simulink model "model"  (R2021a)
settings: Solver=VariableStepAuto  StartTime=0.0  StopTime=11  RelTol=1e-3
values from neighbouring files (symbols this model uses):
  b = .071    (= 0.071)    [main.m]
  Ipn = 2    [main.m]
  J = 21890.7e-6    (= 0.0218907)    [main.m]
  K = .573    (= 0.573)    [main.m]
  L = 5.4e-3    (= 0.0054)    [main.m]
  M = 171    [main.m]
  phi_max = 10    [main.m]
  R = 1.45    [main.m]
  Ts = 0.001    [main.m]
  U = 48    [main.m]
  U_I_max = 4    [main.m]
libraries: simulink x5, pid_lib x2, spsPWMGeneratorDCDCLib x1, eeQuadratureDecoder x1
settings Model: Creator=artof  LastModifiedBy=artof
settings SolverCC: AlgebraicLoopSolver=TrustRegion
settings DebuggingCC: SFMachineParentedDataDiag=warning

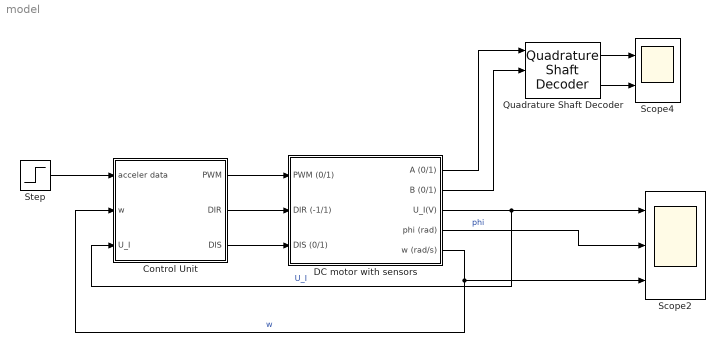
== system model ==
  Control Unit : Subsystem
  DC motor with sensors : Subsystem
  Quadrature Shaft Decoder : eeQuadratureDecoder/Quadrature Shaft Decoder  NPulse=4  Ts=Ts
      settings: SourceProductBaseCode=PS
  Scope2 : Scope  NumInputPorts=3
  Scope4 : Scope  NumInputPorts=2
  Step : Step  After=9.81  SampleTime=0
  wires:
  DC motor with sensors/1(A (0/1)) -> Quadrature Shaft Decoder/1
  DC motor with sensors/2(B (0/1)) -> Quadrature Shaft Decoder/2
  DC motor with sensors/5(w (rad/s)) -> Control Unit/2(w), Scope2/3  "w"
  DC motor with sensors/4(phi (rad)) -> Scope2/2  "phi"
  DC motor with sensors/3(U_I(V)) -> Scope2/1, Control Unit/3(U_I)  "U_I"
  Control Unit/1(PWM) -> DC motor with sensors/1(PWM (0/1))
  Control Unit/2(DIR) -> DC motor with sensors/2(DIR (-1/1))
  Control Unit/3(DIS) -> DC motor with sensors/3(DIS (0/1))
  Quadrature Shaft Decoder/1 -> Scope4/1
  Quadrature Shaft Decoder/2 -> Scope4/2
  Step/1 -> Control Unit/1(acceler data)

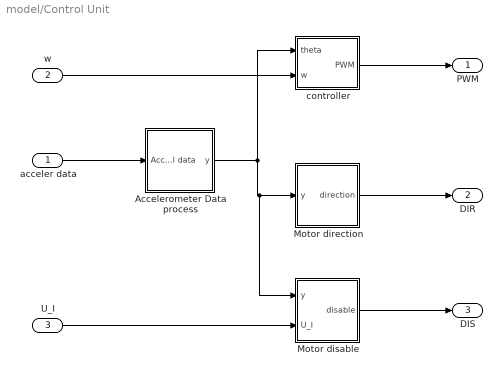
== system model/Control Unit ==
  acceler data : Inport
  w : Inport  Port=2
  U_I : Inport  Port=3
  Accelerometer Data process : Subsystem
  Motor direction : Subsystem
  Motor disable : Subsystem
  controller : Subsystem
  PWM : Outport
  DIR : Outport  Port=2
  DIS : Outport  Port=3
  wires:
  Accelerometer Data process/1(y) -> controller/1(theta), Motor disable/1(y), Motor direction/1(y)
  acceler data/1 -> Accelerometer Data process/1(Accel data)
  Motor direction/1(direction) -> DIR/1
  w/1 -> controller/2(w)
  controller/1(PWM) -> PWM/1
  U_I/1 -> Motor disable/2(U_I)
  Motor disable/1(disable) -> DIS/1

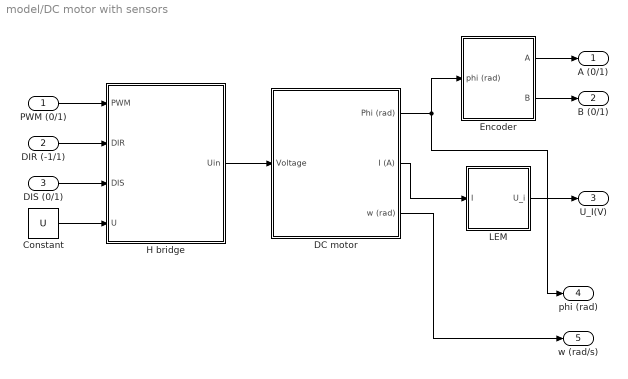
== system model/DC motor with sensors ==
  PWM (0/1) : Inport
  DIR (-1/1) : Inport  Port=2
  DIS (0/1) : Inport  Port=3
  Constant : Constant  Value=U
  DC motor : Subsystem
  Encoder : Subsystem
  H bridge : Subsystem
  LEM : Subsystem
  A (0/1) : Outport
  B (0/1) : Outport  Port=2
  U_I(V) : Outport  Port=3
  phi (rad) : Outport  Port=4
  w (rad/s) : Outport  Port=5
  wires:
  PWM (0/1)/1 -> H bridge/1(PWM)
  DIR (-1/1)/1 -> H bridge/2(DIR)
  H bridge/1(Uin) -> DC motor/1("Voltage ")
  DC motor/1(Phi (rad)) -> Encoder/1(phi (rad)), phi (rad)/1
  Encoder/2(B) -> B (0/1)/1
  Constant/1 -> H bridge/4(U)
  DC motor/2(I (A)) -> LEM/1(I)
  Encoder/1(A) -> A (0/1)/1
  LEM/1(U_i) -> U_I(V)/1
  DIS (0/1)/1 -> H bridge/3(DIS)
  DC motor/3(w (rad)) -> w (rad/s)/1

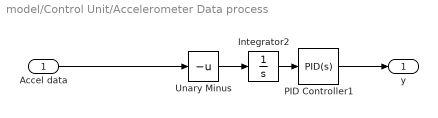
== system model/Control Unit/Accelerometer Data process ==
  Accel data : Inport
  Integrator2 : Integrator
  PID Controller1 : pid_lib/PID Controller  Controller=PID  Form=Parallel  TimeDomain=Continuous-time  UseExternalTs=off  SampleTime=-1  IntegratorMethod=Forward Euler  FilterMethod=Forward Euler  ControllerParametersSource=internal  P=1  I=0.1  D=0  UseFilter=on  N=100  TunerSelectOption=Transfer Function Based (PID Tuner App)  InitialConditionSource=internal  InitialConditionForIntegrator=0  InitialConditionForFilter=0  DifferentiatorICPrevScaledInput=0  ExternalReset=none  TrackingMode=off  Kt=1  LimitOutput=off  SatLimitsSource=internal  UpperSaturationLimit=inf  LowerSaturationLimit=-inf  LinearizeAsGain=on  AntiWindupMode=none  Kb=1  POutMin=[]  POutMax=[]  IOutMin=[]  IOutMax=[]  DOutMin=[]  DOutMax=[]  NOutMin=[]  NOutMax=[]  SumOutMin=[]  SumOutMax=[]  SaturationOutMin=[]  SaturationOutMax=[]  PParamMin=[]  PParamMax=[]  IParamMin=[]  IParamMax=[]  DParamMin=[]  DParamMax=[]  NParamMin=[]  NParamMax=[]  KbParamMin=[]  KbParamMax=[]  KtParamMin=[]  KtParamMax=[]  KbOutMin=[]  KbOutMax=[]  KtOutMin=[]  KtOutMax=[]  IntegratorOutMin=[]  IntegratorOutMax=[]  FilterOutMin=[]  FilterOutMax=[]  SumI1OutMin=[]  SumI1OutMax=[]  SumI2OutMin=[]  SumI2OutMax=[]  SumI3OutMin=[]  SumI3OutMax=[]  SumI4OutMin=[]  SumI4OutMax=[]  SumDOutMin=[]  SumDOutMax=[]  DifferentiatorOutMin=[]  DifferentiatorOutMax=[]  FilterDiffOutCoefMin=[]  FilterDiffOutCoefMax=[]  ReciprocalOutMin=[]  ReciprocalOutMax=[]  SumDenOutMin=[]  SumDenOutMax=[]  SumNumOutMin=[]  SumNumOutMax=[]  DivideOutMin=[]  DivideOutMax=[]  UdiffTsProdOutMin=[]  UdiffTsProdOutMax=[]  NTsProdOutMin=[]  NTsProdOutMax=[]  UintegralTsProdOutMin=[]  UintegralTsProdOutMax=[]  UngainTsProdOutMin=[]  UngainTsProdOutMax=[]  IntegratorContinuousStateAttributes=''  IntegratorStateMustResolveToSignalObject=off  IntegratorRTWStateStorageClass=Auto  FilterContinuousStateAttributes=''  FilterStateMustResolveToSignalObject=off  FilterRTWStateStorageClass=Auto  ParallelPVariant=InternalParameters  IdealPVariant=Disabled  IVariant=InternalParameters  DVariant=InternalParameters  IntegratorVariant=Continuous  SatVariant=Disabled  AWVariant=Passthrough  PCopyVariant=Disabled  TRVariant=Disabled  FdbkBlocksVariant=Forward  IdealPFdbkVariant=Disabled  SatFdbkVariant=Disabled  DerivativeFilterVariant=ContFilter  NVariant=InternalParameters  NCopyVariant=Disabled  FilterICVariant=InternalICsFilter  IntegratorICVariant=InternalICs  ExternalResetVariant=Disabled  TRSumVariant=Passthrough  SumFdbkVariant=Disabled  SumVariant=Sum_PID  TsampFilterVariant=InternalTs  TsampNgainVariant=Passthrough  TsampIntegralVariant=Passthrough  ExternalSaturationOutDataTypeStr=Inherit: Same as second input
  Unary Minus : UnaryMinus
  y : Outport
  wires:
  Integrator2/1 -> PID Controller1/1
  PID Controller1/1 -> y/1
  Unary Minus/1 -> Integrator2/1
  Accel data/1 -> Unary Minus/1

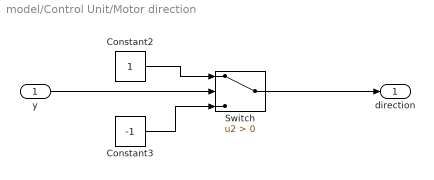
== system model/Control Unit/Motor direction ==
  y : Inport
  Constant2 : Constant
  Constant3 : Constant  Value=-1
  Switch : Switch  Criteria=u2 > Threshold
  direction : Outport
  wires:
  Constant3/1 -> Switch/3
  Switch/1 -> direction/1
  Constant2/1 -> Switch/1
  y/1 -> Switch/2

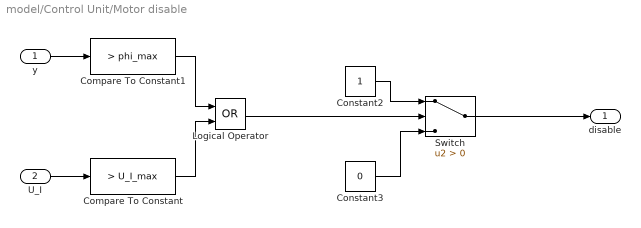
== system model/Control Unit/Motor disable ==
  y : Inport
  U_I : Inport  Port=2
  Compare To Constant : simulink/Logic and Bit Operations/Compare To Constant  relop=>  const=U_I_max  OutDataTypeStr=boolean
  Compare To Constant1 : simulink/Logic and Bit Operations/Compare To Constant  relop=>  const=phi_max  OutDataTypeStr=boolean
  Constant2 : Constant
  Constant3 : Constant  Value=0
  Logical Operator : Logic  Operator=OR  AllPortsSameDT=off  OutDataTypeStr=boolean
  Switch : Switch  Criteria=u2 > Threshold
  disable : Outport
  wires:
  Constant2/1 -> Switch/1
  Switch/1 -> disable/1
  Constant3/1 -> Switch/3
  U_I/1 -> Compare To Constant/1
  Compare To Constant/1 -> Logical Operator/2
  y/1 -> Compare To Constant1/1
  Compare To Constant1/1 -> Logical Operator/1
  Logical Operator/1 -> Switch/2

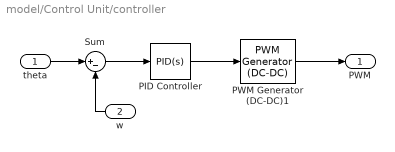
== system model/Control Unit/controller ==
  theta : Inport
  w : Inport  Port=2
  PID Controller : pid_lib/PID Controller  Controller=PID  Form=Parallel  TimeDomain=Continuous-time  UseExternalTs=off  SampleTime=-1  IntegratorMethod=Forward Euler  FilterMethod=Forward Euler  ControllerParametersSource=internal  P=100  I=0.1  D=0.001  UseFilter=on  N=100  TunerSelectOption=Transfer Function Based (PID Tuner App)  InitialConditionSource=internal  InitialConditionForIntegrator=0  InitialConditionForFilter=0  DifferentiatorICPrevScaledInput=0  ExternalReset=none  TrackingMode=off  Kt=1  LimitOutput=on  SatLimitsSource=internal  UpperSaturationLimit=1  LowerSaturationLimit=0  LinearizeAsGain=on  AntiWindupMode=none  Kb=1  POutMin=[]  POutMax=[]  IOutMin=[]  IOutMax=[]  DOutMin=[]  DOutMax=[]  NOutMin=[]  NOutMax=[]  SumOutMin=[]  SumOutMax=[]  SaturationOutMin=[]  SaturationOutMax=[]  PParamMin=[]  PParamMax=[]  IParamMin=[]  IParamMax=[]  DParamMin=[]  DParamMax=[]  NParamMin=[]  NParamMax=[]  KbParamMin=[]  KbParamMax=[]  KtParamMin=[]  KtParamMax=[]  KbOutMin=[]  KbOutMax=[]  KtOutMin=[]  KtOutMax=[]  IntegratorOutMin=[]  IntegratorOutMax=[]  FilterOutMin=[]  FilterOutMax=[]  SumI1OutMin=[]  SumI1OutMax=[]  SumI2OutMin=[]  SumI2OutMax=[]  SumI3OutMin=[]  SumI3OutMax=[]  SumI4OutMin=[]  SumI4OutMax=[]  SumDOutMin=[]  SumDOutMax=[]  DifferentiatorOutMin=[]  DifferentiatorOutMax=[]  FilterDiffOutCoefMin=[]  FilterDiffOutCoefMax=[]  ReciprocalOutMin=[]  ReciprocalOutMax=[]  SumDenOutMin=[]  SumDenOutMax=[]  SumNumOutMin=[]  SumNumOutMax=[]  DivideOutMin=[]  DivideOutMax=[]  UdiffTsProdOutMin=[]  UdiffTsProdOutMax=[]  NTsProdOutMin=[]  NTsProdOutMax=[]  UintegralTsProdOutMin=[]  UintegralTsProdOutMax=[]  UngainTsProdOutMin=[]  UngainTsProdOutMax=[]  IntegratorContinuousStateAttributes=''  IntegratorStateMustResolveToSignalObject=off  IntegratorRTWStateStorageClass=Auto  FilterContinuousStateAttributes=''  FilterStateMustResolveToSignalObject=off  FilterRTWStateStorageClass=Auto  ParallelPVariant=InternalParameters  IdealPVariant=Disabled  IVariant=InternalParameters  DVariant=InternalParameters  IntegratorVariant=Continuous  SatVariant=Enabled  AWVariant=Passthrough  PCopyVariant=Disabled  TRVariant=Disabled  FdbkBlocksVariant=Forward  IdealPFdbkVariant=Disabled  SatFdbkVariant=Disabled  DerivativeFilterVariant=ContFilter  NVariant=InternalParameters  NCopyVariant=Disabled  FilterICVariant=InternalICsFilter  IntegratorICVariant=InternalICs  ExternalResetVariant=Disabled  TRSumVariant=Passthrough  SumFdbkVariant=Disabled  SumVariant=Sum_PID  TsampFilterVariant=InternalTs  TsampNgainVariant=Passthrough  TsampIntegralVariant=Passthrough  ExternalSaturationOutDataTypeStr=Inherit: Same as second input
  PWM Generator (DC-DC)1 : spsPWMGeneratorDCDCLib/PWM Generator (DC-DC)  Fsw=freq  Ts=0
  Sum : Sum  Inputs=|+-
  PWM : Outport
  wires:
  theta/1 -> Sum/1
  w/1 -> Sum/2
  PWM Generator (DC-DC)1/1 -> PWM/1
  PID Controller/1 -> PWM Generator (DC-DC)1/1
  Sum/1 -> PID Controller/1

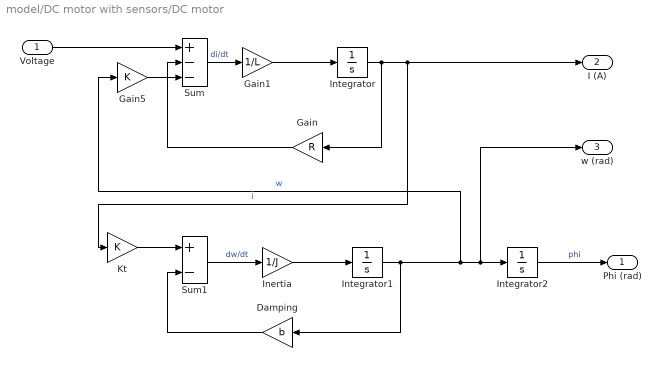
== system model/DC motor with sensors/DC motor ==
  "Voltage " : Inport
  Damping : Gain  Gain=b
  Gain : Gain  Gain=R
  Gain1 : Gain  Gain=1/L
  Gain5 : Gain  Gain=K
  Inertia : Gain  Gain=1/J
  Integrator : Integrator
  Integrator1 : Integrator
  Integrator2 : Integrator
  Kt : Gain  Gain=K
  Sum : Sum  Inputs=+--
  Sum1 : Sum  Inputs=+-
  Phi (rad) : Outport
  I (A) : Outport  Port=2
  w (rad) : Outport  Port=3
  wires:
  Integrator2/1 -> Phi (rad)/1  "phi"
  Gain1/1 -> Integrator/1
  Gain5/1 -> Sum/3
  Inertia/1 -> Integrator1/1
  "Voltage "/1 -> Sum/1
  Integrator/1 -> Gain/1, I (A)/1, Kt/1  "i"
  Integrator1/1 -> Damping/1, w (rad)/1, Integrator2/1, Gain5/1  "w"
  Damping/1 -> Sum1/2
  Sum/1 -> Gain1/1  "di/dt"
  Kt/1 -> Sum1/1
  Gain/1 -> Sum/2
  Sum1/1 -> Inertia/1  "dw/dt"

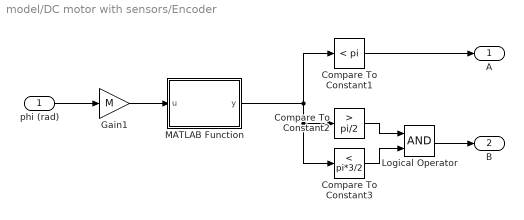
== system model/DC motor with sensors/Encoder ==
  phi (rad) : Inport
  Compare To Constant1 : simulink/Logic and Bit Operations/Compare To Constant  relop=<  const=pi  OutDataTypeStr=boolean
  Compare To Constant2 : simulink/Logic and Bit Operations/Compare To Constant  relop=>  const=pi/2  OutDataTypeStr=boolean
  Compare To Constant3 : simulink/Logic and Bit Operations/Compare To Constant  relop=<  const=pi*3/2  OutDataTypeStr=boolean
  Gain1 : Gain  Gain=M
  Logical Operator : Logic  AllPortsSameDT=off  OutDataTypeStr=boolean
  MATLAB Function : MATLAB Function  TreatAsAtomicUnit=on
  A : Outport
  B : Outport  Port=2
  wires:
  phi (rad)/1 -> Gain1/1
  Compare To Constant1/1 -> A/1
  Compare To Constant2/1 -> Logical Operator/1
  Logical Operator/1 -> B/1
  Gain1/1 -> MATLAB Function/1(u)
  MATLAB Function/1(y) -> Compare To Constant1/1, Compare To Constant3/1, Compare To Constant2/1
  Compare To Constant3/1 -> Logical Operator/2

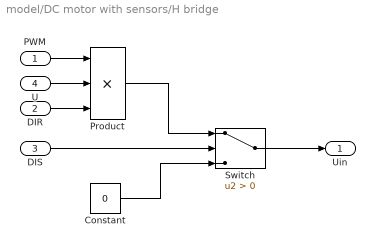
== system model/DC motor with sensors/H bridge ==
  PWM : Inport
  DIR : Inport  Port=2
  DIS : Inport  Port=3
  U : Inport  Port=4
  Constant : Constant  Value=0
  Product : Product  Inputs=3
  Switch : Switch  Criteria=u2 > Threshold
  Uin : Outport
  wires:
  U/1 -> Product/2
  PWM/1 -> Product/1
  DIS/1 -> Switch/2
  Constant/1 -> Switch/3
  Switch/1 -> Uin/1
  Product/1 -> Switch/1
  DIR/1 -> Product/3

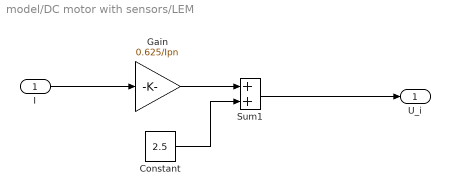
== system model/DC motor with sensors/LEM ==
  I : Inport
  Constant : Constant  Value=2.5
  Gain : Gain  Gain=0.625/Ipn
  Sum1 : Sum
  U_i : Outport
  wires:
  Gain/1 -> Sum1/1
  Sum1/1 -> U_i/1
  Constant/1 -> Sum1/2
  I/1 -> Gain/1

== matlab function model/DC motor with sensors/Encoder/MATLAB Function ==
  data: u input; y output
function y = fcn(u)
y = mod(u,2*pi);
